simulink model "f_validation_V1_19b"  (R2019b)
settings: Solver=ode4  StartTime=0.0  StopTime=104  FixedStep=0.01  RelTol=1e-3
model workspace (MAT data in the model file):
  x2xx = 0
values from neighbouring files (symbols this model uses):
  KDspd = 0    [frequency_validation.m]
  KIspd = 0    [frequency_validation.m]
  KPspd = 20    [frequency_validation.m]
  PARSa = [ ... (first row only)    [Q_ART_par.m]
  PARSu = zeros(Nu,5)    [Q_ART_par.m]
  Q0 = zeros(Nu+2,1)    [frequency_validation.m]
  QD0 = Q0    [frequency_validation.m]
  v_ref = vconst    (= 5.55555555556)    [frequency_validation.m]
undefined symbols (not defined in the file or in its folder): axle_rate_limit, Lspd, Nspd, Tmc, Uspd
libraries: simulink x2
(part 2 of 3)

== matlab function f_validation_V1_19b/time-domain-test/single-funky-sattyre-nonlinear-variable-crrc/V_tyre ==
  data: q input; Vaa output; qd input
function Vaa = calculate_v_tyre(q, qd)

%%%%%%%%%%%%%%%%%%%%%%%%%%%%%%%%%%%%%%%%%%%%%%%%%%%%%%%%%%%%%%%%%%%%%%%%%
Va = zeros(2, 8); % axle velocities in globals
Vj = zeros(2, 4); % joint velocities in globals
Vaa = Va; % axle velocities in locals
%%%%%%%%%%%%%%%%%%%%%%%%%%%%%%%%%%%%%%%%%%%%%%%%%%%%%%%%%%%%%%%%%%%%%%%%%%
% Parameter given
% M J L xg = mass, moment of inertia, length, cg location measured from rear joint

LL = [11.4, 9.4, 11.4]';
XG = [5.538, 4.757, 11.4 - 5.538]';
XA = [8.9, 7.4, 1.5, 7.9, 1.5, 9.9, 4.0, 2.5]';
KK = [1, 1, 1, 2, 2, 3, 3, 3]';
%%%%%%%%%%%%%%%%%%%%%%%%%%%%%%%%%%%%%%%%%%%%%%%%%%%%%%%%%%%%%%%%%%%%%%%%%%
% Rotation matrix

uu = zeros(2, 3); 
nn = zeros(2, 3); 
for i = 1:3
    c = cos(q(i + 2));
    s = sin(q(i + 2)); 
    uu(:, i) = [c, s]';
    nn(:, i) = [-s, c]';
end
%%%%%%%%%%%%%%%%%%%%%%%%%%%%%%%%%%%%%%%%%%%%%%%%%%%%%%%%%%%%%%%%%%%%%%%%%%
% % from first unit cg to first virtual joint
% 
% l = 11.4;
% b1 = 5.538;
% 
% q = zeros(5,1);
% q(1) = q(1) + (l - b1) * cos(q(3));
% q(2) = q(2) + (l - b1) * sin(q(3));
% 
% qd = zeros(5,1);
% qd(1) = qd(1) + (l - b1) * qd(3) * sin(q(3));
% qd(2) = qd(2) - (l - b1) * qd(3) * cos(q(3));
%%%%%%%%%%%%%%%%%%%%%%%%%%%%%%%%%%%%%%%%%%%%%%%%%%%%%%%%%%%%%%%%%%%%%%%%%%
% calculate v_tyre

Vj(:, 1) = [qd(1), qd(2)]';

for i = 1:3
    Vj(:, i+1) = Vj(:, i) - qd(i + 2) * LL(i) * nn(:, i);
end

for i = 1:8
    Va(:, i) = Vj(:, KK(i) + 1) + qd(KK(i) + 2) * XA(i) * nn(:, KK(i));
    Vax = dot(Va(:, i), uu(:, KK(i)));
    Vay = dot(Va(:, i), nn(:, KK(i)));
    Vaa(:, i) = [Vax; Vay];
end
%%%%%%%%%%%%%%%%%%%%%%%%%%%%%%%%%%%%%%%%%%%%%%%%%%%%%%%%%%%%%%%%%%%%%%%%%%

== matlab function f_validation_V1_19b/time-domain-test/single-general-lineartyre-nonlinear-variable-crrc/qdd ==
  data: M input; C input; Q input; qdd output
function qdd = calculate_qdd(M, C, Q)

qdd = inv(M)*(Q - C);

end

== matlab function f_validation_V1_19b/time-domain-test/single-funky-sattyre-nonlinear-variable-crrc/Fy from slip ==
  data: Alpha output; Steer input; V_tyre input; Fy output
function [Alpha, Fy] = LatForce(Steer, V_tyre)

small = 1e-4;
deg = pi/180;
Fy = zeros(8, 1); 
Alpha = zeros(8, 1); 
Ca = 3065 * 180 / pi;
Sat = Ca * 10 * deg; 

for i = 1:8
    vx = V_tyre(1, i) * cos(Steer(i)) + V_tyre(2, i) * sin(Steer(i));
    vy = -V_tyre(1, i) * sin(Steer(i)) + V_tyre(2, i) * cos(Steer(i));
    if abs(vx) < small
        if abs(vy) < small
            alpha = 0;
            fy = 0.0;
        else
            alpha = 90;
            fy = -Sat * sign(vy);
        end
    else
        alpha = atan2(vy, vx);
        fy = abs(Ca * alpha);
        fy = min(Sat, fy);
        fy = -fy * sign(vy);
    end
    Fy(i) = fy;
    Alpha(i) = alpha;
end

== matlab function f_validation_V1_19b/time-domain-test/double-general-lineartyre-nonlinear-variable-matrix/C ==
  data: q input; qd input; C output
function C = calculate_C(q, qd)

m1 = 11142;
m3 = 11142;
m2 = 7651; 
l_j1j2 = 11.4;
l_j2j3 = 9.4;
l_j1g1 = 5.862; 
l_j2g2 = 4.643; 
l_j3g3 = 5.538; 

psi1 = q(3);
psi2 = q(4);
psi3 = q(5);
xd = qd(1);
yd = qd(2);
psi1d = qd(3);
psi2d = qd(4);
psi3d = qd(5);

C = [0, 0, (l_j1g1*m1 + l_j1j2*(m2 + m3))*cos(psi1)*psi1d, (l_j2g2*m2 + l_j2j3*m3)*cos(psi2)*psi2d, l_j3g3*m3*cos(psi3)*psi3d;
     0, 0, (l_j1g1*m1 + l_j1j2*(m2 + m3))*sin(psi1)*psi1d, (l_j2g2*m2 + l_j2j3*m3)*sin(psi2)*psi2d, l_j3g3*m3*sin(psi3)*psi3d;
     1/2*(l_j1g1*m1 + l_j1j2*(m2 + m3))*cos(psi1)*psi1d, 1/2*(l_j1g1*m1 + l_j1j2*(m2 + m3))*sin(psi1)*psi1d, -1/2*(l_j1g1*m1 + l_j1j2*(m2 + m3))*(xd*cos(psi1)+yd*sin(psi1))+1/2*(l_j2g2*l_j1j2*m2+l_j1j2*l_j2j3*m3)*sin(psi1-psi2)*psi2d+1/2*l_j3g3*l_j1j2*m3*sin(psi1-psi3)*psi3d, (l_j2g2*l_j1j2*m2+l_j1j2*l_j2j3*m3)*sin(psi1-psi2)*(-1/2*psi1d+psi2d), l_j3g3*l_j1j2*m3*sin(psi1-psi3)*(-1/2*psi1d+psi3d);
     1/2*(l_j2g2*m2 + l_j2j3*m3)*cos(psi2)*psi2d, 1/2*(l_j2g2*m2 + l_j2j3*m3)*sin(psi2)*psi2d, (l_j2g2*l_j1j2*m2+l_j1j2*l_j2j3*m3)*sin(psi1-psi2)*(-psi1d+1/2*psi2d), -1/2*(l_j2g2*m2+l_j2j3*m3)*(xd*cos(psi2)+yd*sin(psi2))-1/2*(l_j2g2*l_j1j2*m2+l_j1j2*l_j2j3*m3)*sin(psi1-psi2)*psi1d+1/2*l_j3g3*l_j2j3*m3*sin(psi2-psi3)*psi3d, l_j3g3*l_j2j3*m3*sin(psi2-psi3)*(-1/2*psi2d+psi3d);
     1/2*l_j3g3*m3*cos(psi3)*psi3d, 1/2*l_j3g3*m3*sin(psi3)*psi3d, l_j3g3*l_j1j2*m3*sin(psi1-psi3)*(-psi1d+1/2*psi3d), l_j3g3*l_j2j3*m3*sin(psi2-psi3)*(-psi2d+1/2*psi3d), -1/2*l_j3g3*m3*(xd*cos(psi3)+yd*sin(psi3))-1/2*l_j3g3*l_j1j2*m3*sin(psi1-psi3)*psi1d-1/2*l_j3g3*l_j2j3*m3*sin(psi2-psi3)*psi2d;];

end

== matlab function f_validation_V1_19b/time-domain-test/double-general-lineartyre-nonlinear-variable-matrix/D ==
  data: D output
function D = calculate_D()

d1 = 10000;
d2 = 10000;

delta_kj = eye(3);
dj = [0, d1, d2, 0]';
D = zeros(5);

for k = 1:5
    for l = 1:5
        if k > 2 && l > 2
            if  l == k
                D(k, l) = (1 - delta_kj(1, k-2))*dj(k - 2) + (1 - delta_kj(3, k-2))*dj(k - 1);
            elseif l == k-1
                D(k, l) = -(1 - delta_kj(1, k-2))*dj(k - 2);
            elseif l == k+1
                D(k, l) = -(1 - delta_kj(3, k-2))*dj(k - 1);
            else
                D(k, l) = 0;
            end
        end
    end
end

end

== matlab function f_validation_V1_19b/time-domain-test/double-general-lineartyre-nonlinear-variable-matrix1/qdd ==
  data: M input; C input; D input; qd input; Q input; qdd output
function qdd = calculate_qdd(M, C, D, qd, Q)

qdd = inv(M)*(Q - C * qd - D * qd);

end

== matlab function f_validation_V1_19b/time-domain-test/double-general-lineartyre-nonlinear-variable-matrix/M ==
  data: M output; q input
function M = calculate_M(q)

psi1 = q(3);
psi2 = q(4);
psi3 = q(5);

m1 = 11142;
m3 = 11142;
m2 = 7651; 
l_j1j2 = 11.4;
l_j2j3 = 9.4;
l_j1g1 = 5.862; 
l_j2g2 = 4.643; 
l_j3g3 = 5.538; 
iz1 = 143570; 
iz3 = 143570; 
iz2 = 37800;

l_kj = [l_j1g1, l_j1j2, l_j1j2;
             0, l_j2g2, l_j2j3;
             0,      0, l_j3g3;];
delta_kj = eye(3);
Jc = zeros(3, 5, 3);
for j = 1:3
    Jc(:, :, j) = [1, 0,  l_kj(1, j) * sin(psi1),  l_kj(2, j) * sin(psi2),  l_kj(3, j) * sin(psi3);
          0, 1, -l_kj(1, j) * cos(psi1), -l_kj(2, j) * cos(psi2), -l_kj(3, j) * cos(psi3);
          0, 0,          delta_kj(1, j),          delta_kj(2, j),          delta_kj(3, j);];
end

mj = [m1, m2, m3]';
izj = [iz1, iz2, iz3]';
Mj = zeros(3, 3, 3);
for j = 1:3
    Mj(:, :, j) = diag([mj(j), mj(j), izj(j)]);
end

M = zeros(5, 5);
for j = 1:3
    M = M + Jc(:, :, j)' * Mj(:, :, j) * Jc(:, :, j);
end

end

== matlab function f_validation_V1_19b/time-domain-test/double-general-lineartyre-nonlinear-variable-matrix/Tau_tire ==
  data: q input; qd input; delta input; Fx input; Tau_tire output; Alpha output
function [Tau_tire, Alpha] = calculate_Tau_tire(q, qd, delta, Fx)

% coefficient

l_j1j2 = 11.4;
l_j2j3 = 9.4;
l_j1a1 = 2.5;
l_j1a2 = 4;
l_j1a3 = 9.9;
l_j2a4 = 1.5;
l_j2a5 = 7.9;
l_j3a6 = 1.5;
l_j3a7 = 7.4;
l_j3a8 = 8.9;
h11 = 0.9625;
h12 = 0.9625;
h13 = 0.98;
h21 = 0.98; 
h22 = 0.98;
h31 = 0.98;
h32 = 0.9625;
h33 = 0.9625;
ca1 = 3065 * 180 / pi;
ca2 = 3065 * 180 / pi;
ca3 = 3065 * 180 / pi;
ca4 = 3065 * 180 / pi;
ca5 = 3065 * 180 / pi;
ca6 = 3065 * 180 / pi;
ca7 = 3065 * 180 / pi;
ca8 = 3065 * 180 / pi;

x = q(1);
y = q(2);
psi1 = q(3);
psi2 = q(4);
psi3 = q(5);
xd = qd(1);
yd = qd(2);
psi1d = qd(3);
psi2d = qd(4);
psi3d = qd(5);

psij = [psi1, psi2, psi3]';
Rot_w2v = zeros(2, 2, 3);
for i = 1:3
    Rot_w2v(:, :, i) = [cos(psij(i)), -sin(psij(i));
                        sin(psij(i)), cos(psij(i));];
end

Rot_v2t = zeros(2, 2, 8);
for i = 1:8
    Rot_v2t(:, :, i) = [cos(delta(i)), -sin(delta(i));
                        sin(delta(i)), cos(delta(i));];
end

xj = zeros(3, 1);
yj = zeros(3, 1);
xj(1) = x;
yj(1) = y;
xj(2) = x - l_j1j2*cos(psi1);
yj(2) = y - l_j1j2*sin(psi1);
xj(3) = x - l_j1j2*cos(psi1) - l_j2j3*cos(psi2);
yj(3) = y - l_j1j2*sin(psi1) - l_j2j3*sin(psi2);

u = zeros(2, 3);
n = zeros(2, 3);
for i = 1:3
    u(:, i)=[cos(q(i + 2)), sin(q(i + 2))]';
    n(:, i)=[-sin(q(i + 2)), cos(q(i + 2))]';
end

IU = [1, 1, 1, 2, 2, 3, 3, 3]';
l_ja = [l_j1a1, l_j1a2, l_j1a3, l_j2a4, l_j2a5, l_j3a6, l_j3a7, l_j3a8]';
ha = [h11, h12, h13, h21, h22, h31, h32, h33]';

L_long1 = [cos(psi1), cos(psi1), cos(psi1), cos(psi2), cos(psi2), cos(psi3), cos(psi3), cos(psi3);
           sin(psi1), sin(psi1), sin(psi1), sin(psi2), sin(psi2), sin(psi3), sin(psi3), sin(psi3);
           -h11, -h12, -h13, l_j1j2*sin(psi1-psi2), l_j1j2*sin(psi1-psi2), l_j1j2*sin(psi1-psi3), l_j1j2*sin(psi1-psi3), l_j1j2*sin(psi1-psi3);
           0, 0, 0, -h21, -h22, l_j2j3*sin(psi2-psi3), l_j2j3*sin(psi2-psi3), l_j2j3*sin(psi2-psi3);
           0, 0, 0, 0, 0, -h31, -h32, -h33;];

L_long2 = [cos(psi1), cos(psi1), cos(psi1), cos(psi2), cos(psi2), cos(psi3), cos(psi3), cos(psi3);
           sin(psi1), sin(psi1), sin(psi1), sin(psi2), sin(psi2), sin(psi3), sin(psi3), sin(psi3);
           h11, h12, h13, l_j1j2*sin(psi1-psi2), l_j1j2*sin(psi1-psi2), l_j1j2*sin(psi1-psi3), l_j1j2*sin(psi1-psi3), l_j1j2*sin(psi1-psi3);
           0, 0, 0, h21, h22, l_j2j3*sin(psi2-psi3), l_j2j3*sin(psi2-psi3), l_j2j3*sin(psi2-psi3);
           0, 0, 0, 0, 0, h31, h32, h33;];

L_lat1 = [-sin(psi1), -sin(psi1), -sin(psi1), -sin(psi2), -sin(psi2), -sin(psi3), -sin(psi3), -sin(psi3);
          cos(psi1), cos(psi1), cos(psi1), cos(psi2), cos(psi2), cos(psi3), cos(psi3), cos(psi3);
          -l_j1a1, -l_j1a2, -l_j1a3, -l_j1j2*cos(psi1-psi2), -l_j1j2*cos(psi1-psi2), -l_j1j2*cos(psi1-psi3), -l_j1j2*cos(psi1-psi3), -l_j1j2*cos(psi1-psi3);
          0, 0, 0, -l_j2a4, -l_j2a5, -l_j2j3*cos(psi2-psi3), -l_j2j3*cos(psi2-psi3), -l_j2j3*cos(psi2-psi3);
          0, 0, 0, 0, 0, -l_j3a6, -l_j3a7, -l_j3a8;];

L_lat2 = [-sin(psi1), -sin(psi1), -sin(psi1), -sin(psi2), -sin(psi2), -sin(psi3), -sin(psi3), -sin(psi3);
          cos(psi1), cos(psi1), cos(psi1), cos(psi2), cos(psi2), cos(psi3), cos(psi3), cos(psi3);
          -l_j1a1, -l_j1a2, -l_j1a3, -l_j1j2*cos(psi1-psi2), -l_j1j2*cos(psi1-psi2), -l_j1j2*cos(psi1-psi3), -l_j1j2*cos(psi1-psi3), -l_j1j2*cos(psi1-psi3);
          0, 0, 0, -l_j2a4, -l_j2a5, -l_j2j3*cos(psi2-psi3), -l_j2j3*cos(psi2-psi3), -l_j2j3*cos(psi2-psi3);
          0, 0, 0, 0, 0, -l_j3a6, -l_j3a7, -l_j3a8;];

Delta_c = zeros(8, 8);
Delta_s = zeros(8, 8);
for i = 1:8
    Delta_c(i, i) = cos(delta(i));
    Delta_s(i, i) = sin(delta(i));
end

vxj = zeros(3, 1);
vyj = zeros(3, 1);
vxj(1) = xd;
vyj(1) = yd;
vxj(2) = xd + l_j1j2*sin(psi1)*psi1d;
vyj(2) = yd - l_j1j2*cos(psi1)*psi1d;
vxj(3) = xd + l_j1j2*sin(psi1)*psi1d + l_j2j3*sin(psi2)*psi2d;
vyj(3) = yd - l_j1j2*cos(psi1)*psi1d - l_j2j3*cos(psi2)*psi2d;
va1 = zeros(2, 8);
va2 = zeros(2, 8);
psidj = [psi1d, psi2d, psi3d]';
for i = 1:8
    va1(:, i) = [vxj(IU(i)); vyj(IU(i))] - n(:, IU(i))*l_ja(i)*psidj(IU(i)) + (-1)*u(:, IU(i))*ha(i)*psidj(IU(i));
    va2(:, i) = [vxj(IU(i)); vyj(IU(i))] - n(:, IU(i))*l_ja(i)*psidj(IU(i)) + u(:, IU(i))*ha(i)*psidj(IU(i));
end

va1_v = zeros(2, 8);
va2_v = zeros(2, 8);
for i = 1:8
    va1_v(:, i) = inv(Rot_w2v(:, :, IU(i)))*va1(:, i);
    va2_v(:, i) = inv(Rot_w2v(:, :, IU(i)))*va2(:, i);
end

beta1 = zeros(8, 1);
beta2 = zeros(8, 1);
for i = 1:8
    beta1(i) = atan2(va1_v(2, i), va1_v(1, i));
    beta2(i) = atan2(va2_v(2, i), va2_v(1, i));
end

ca = [ca1, ca2, ca3, ca4, ca5, ca6, ca7, ca8]';
Ca = diag(ca);

Tau_tire = L_long1 * (Delta_c * Fx / 2 - Delta_s * Ca * (delta - beta1)) ...
         + L_long2 * (Delta_c * Fx / 2 - Delta_s * Ca * (delta - beta2)) ...
         + L_lat1 * (Delta_s * Fx / 2 + Delta_c * Ca * (delta - beta1)) ...
         + L_lat2 * (Delta_s * Fx / 2 + Delta_c * Ca * (delta - beta2));

beta = (beta1 + beta2) / 2;
Alpha = delta - beta;

end

== matlab function f_validation_V1_19b/time-domain-test/double-general-lineartyre-nonlinear-variable-matrix/qdd ==
  data: M input; C input; D input; qd input; Q input; qdd output
function qdd = calculate_qdd(M, C, D, qd, Q)

qdd = inv(M)*(Q - C * qd - D * qd);

end

== matlab function f_validation_V1_19b/time-domain-test/single-general-lineartyre-nonlinear-variable-matrix/C ==
  data: q input; qd input; C output
function C = calculate_C(q, qd)

m1 = 11142;
m3 = 11142;
m2 = 7651; 
l_j1j2 = 11.4;
l_j2j3 = 9.4;
l_j1g1 = 5.862; 
l_j2g2 = 4.643; 
l_j3g3 = 5.538; 

psi1 = q(3);
psi2 = q(4);
psi3 = q(5);
xd = qd(1);
yd = qd(2);
psi1d = qd(3);
psi2d = qd(4);
psi3d = qd(5);

C = [0, 0, (l_j1g1*m1 + l_j1j2*(m2 + m3))*cos(psi1)*psi1d, (l_j2g2*m2 + l_j2j3*m3)*cos(psi2)*psi2d, l_j3g3*m3*cos(psi3)*psi3d;
     0, 0, (l_j1g1*m1 + l_j1j2*(m2 + m3))*sin(psi1)*psi1d, (l_j2g2*m2 + l_j2j3*m3)*sin(psi2)*psi2d, l_j3g3*m3*sin(psi3)*psi3d;
     1/2*(l_j1g1*m1 + l_j1j2*(m2 + m3))*cos(psi1)*psi1d, 1/2*(l_j1g1*m1 + l_j1j2*(m2 + m3))*sin(psi1)*psi1d, -1/2*(l_j1g1*m1 + l_j1j2*(m2 + m3))*(xd*cos(psi1)+yd*sin(psi1))+1/2*(l_j2g2*l_j1j2*m2+l_j1j2*l_j2j3*m3)*sin(psi1-psi2)*psi2d+1/2*l_j3g3*l_j1j2*m3*sin(psi1-psi3)*psi3d, (l_j2g2*l_j1j2*m2+l_j1j2*l_j2j3*m3)*sin(psi1-psi2)*(-1/2*psi1d+psi2d), l_j3g3*l_j1j2*m3*sin(psi1-psi3)*(-1/2*psi1d+psi3d);
     1/2*(l_j2g2*m2 + l_j2j3*m3)*cos(psi2)*psi2d, 1/2*(l_j2g2*m2 + l_j2j3*m3)*sin(psi2)*psi2d, (l_j2g2*l_j1j2*m2+l_j1j2*l_j2j3*m3)*sin(psi1-psi2)*(-psi1d+1/2*psi2d), -1/2*(l_j2g2*m2+l_j2j3*m3)*(xd*cos(psi2)+yd*sin(psi2))-1/2*(l_j2g2*l_j1j2*m2+l_j1j2*l_j2j3*m3)*sin(psi1-psi2)*psi1d+1/2*l_j3g3*l_j2j3*m3*sin(psi2-psi3)*psi3d, l_j3g3*l_j2j3*m3*sin(psi2-psi3)*(-1/2*psi2d+psi3d);
     1/2*l_j3g3*m3*cos(psi3)*psi3d, 1/2*l_j3g3*m3*sin(psi3)*psi3d, l_j3g3*l_j1j2*m3*sin(psi1-psi3)*(-psi1d+1/2*psi3d), l_j3g3*l_j2j3*m3*sin(psi2-psi3)*(-psi2d+1/2*psi3d), -1/2*l_j3g3*m3*(xd*cos(psi3)+yd*sin(psi3))-1/2*l_j3g3*l_j1j2*m3*sin(psi1-psi3)*psi1d-1/2*l_j3g3*l_j2j3*m3*sin(psi2-psi3)*psi2d;];

end

== matlab function f_validation_V1_19b/time-domain-test/single-general-lineartyre-nonlinear-variable-matrix/D ==
  data: D output
function D = calculate_D()

d1 = 0;
d2 = 0;

delta_kj = eye(3);
dj = [0, d1, d2, 0]';
D = zeros(5);

for k = 1:5
    for l = 1:5
        if k > 2 && l > 2
            if  l == k
                D(k, l) = (1 - delta_kj(1, k-2))*dj(k - 2) + (1 - delta_kj(3, k-2))*dj(k - 1);
            elseif l == k-1
                D(k, l) = -(1 - delta_kj(1, k-2))*dj(k - 2);
            elseif l == k+1
                D(k, l) = -(1 - delta_kj(3, k-2))*dj(k - 1);
            else
                D(k, l) = 0;
            end
        end
    end
end

end

== matlab function f_validation_V1_19b/time-domain-test/single-general-lineartyre-nonlinear-variable-matrix/M ==
  data: M output; q input
function M = calculate_M(q)

psi1 = q(3);
psi2 = q(4);
psi3 = q(5);

m1 = 11142;
m3 = 11142;
m2 = 7651; 
l_j1j2 = 11.4;
l_j2j3 = 9.4;
l_j1g1 = 5.862; 
l_j2g2 = 4.643; 
l_j3g3 = 5.538; 
iz1 = 143570; 
iz3 = 143570; 
iz2 = 37800;

l_kj = [l_j1g1, l_j1j2, l_j1j2;
             0, l_j2g2, l_j2j3;
             0,      0, l_j3g3;];
delta_kj = eye(3);
Jc = zeros(3, 5, 3);
for j = 1:3
    Jc(:, :, j) = [1, 0,  l_kj(1, j) * sin(psi1),  l_kj(2, j) * sin(psi2),  l_kj(3, j) * sin(psi3);
          0, 1, -l_kj(1, j) * cos(psi1), -l_kj(2, j) * cos(psi2), -l_kj(3, j) * cos(psi3);
          0, 0,          delta_kj(1, j),          delta_kj(2, j),          delta_kj(3, j);];
end

mj = [m1, m2, m3]';
izj = [iz1, iz2, iz3]';
Mj = zeros(3, 3, 3);
for j = 1:3
    Mj(:, :, j) = diag([mj(j), mj(j), izj(j)]);
end

M = zeros(5, 5);
for j = 1:3
    M = M + Jc(:, :, j)' * Mj(:, :, j) * Jc(:, :, j);
end

end

== matlab function f_validation_V1_19b/time-domain-test/single-general-lineartyre-nonlinear-variable-matrix/Tau_tire ==
  data: q input; qd input; delta input; Fx input; Tau_tire output; Alpha output
function [Tau_tire, Alpha] = calculate_Tau_tire(q, qd, delta, Fx)

% coefficient

l_j1j2 = 11.4;
l_j2j3 = 9.4;
l_j1a1 = 2.5;
l_j1a2 = 4;
l_j1a3 = 9.9;
l_j2a4 = 1.5;
l_j2a5 = 7.9;
l_j3a6 = 1.5;
l_j3a7 = 7.4;
l_j3a8 = 8.9;

LL = [l_j1j2, l_j2j3, l_j1j2]';
JA = [l_j1a1, l_j1a2, l_j1a3, l_j2a4, l_j2a5, l_j3a6, l_j3a7, l_j3a8]';
XA = [l_j1j2, l_j1j2, l_j1j2, l_j2j3, l_j2j3, l_j1j2, l_j1j2, l_j1j2]' - JA;
IU = [1, 1, 1, 2, 2, 3, 3, 3]';

Ca = [3065 * 180 / pi, 3065 * 180 / pi, 3065 * 180 / pi, 3065 * 180 / pi, 3065 * 180 / pi, 3065 * 180 / pi, 3065 * 180 / pi, 3065 * 180 / pi]';

uu = zeros(2, 3);
nn = zeros(2, 3);
for i = 1:3
    uu(:, i)=[cos(q(i + 2)), sin(q(i + 2))]';
    nn(:, i)=[-sin(q(i + 2)), cos(q(i + 2))]';
end

psi1 = q(3);
psi2 = q(4);
psi3 = q(5);
xd = qd(1);
yd = qd(2);
psi1d = qd(3);
psi2d = qd(4);
psi3d = qd(5);
psij = [psi1, psi2, psi3]';
l_ja = [l_j1a1, l_j1a2, l_j1a3, l_j2a4, l_j2a5, l_j3a6, l_j3a7, l_j3a8]';

Rot_w2v = zeros(2, 2, 3);
for i = 1:3
    Rot_w2v(:, :, i) = [cos(psij(i)), -sin(psij(i));
                        sin(psij(i)), cos(psij(i));];
end

Rot_v2t = zeros(2, 2, 8);
for i = 1:8
    Rot_v2t(:, :, i) = [cos(delta(i)), -sin(delta(i));
                        sin(delta(i)), cos(delta(i));];
end

vxj = zeros(3, 1);
vyj = zeros(3, 1);
vxj(1) = xd;
vyj(1) = yd;
vxj(2) = xd + l_j1j2*sin(psi1)*psi1d;
vyj(2) = yd - l_j1j2*cos(psi1)*psi1d;
vxj(3) = xd + l_j1j2*sin(psi1)*psi1d + l_j2j3*sin(psi2)*psi2d;
vyj(3) = yd - l_j1j2*cos(psi1)*psi1d - l_j2j3*cos(psi2)*psi2d;
va = zeros(2, 8);
psidj = [psi1d, psi2d, psi3d]';
for i = 1:8
    va(:, i) = [vxj(IU(i)); vyj(IU(i))] - nn(:, IU(i))*l_ja(i)*psidj(IU(i));
end

Va_v = zeros(2, 8);  % axle velocities in locals
for i = 1:8
    Va_v(:, i) = inv(Rot_w2v(:, :, IU(i)))*va(:, i);
end

Fy = zeros(8, 1); 
Alpha = zeros(8, 1); 

beta = zeros(8, 1);
for i = 1:8
    beta(i) = atan2(Va_v(2, i), Va_v(1, i));
end

Vx_t = zeros(8, 1);
Vy_t = zeros(8, 1);
for i = 1:8
    Vx_t(i) = Va_v(1, i) * cos(delta(i)) + Va_v(2, i) * sin(delta(i));
    Vy_t(i) = -Va_v(1, i) * sin(delta(i)) + Va_v(2, i) * cos(delta(i));
end

for i = 1:8
    Alpha(i) = delta(i) - beta(i);
%     Fy(i) = -sign(Vy_t(i)) * Ca(i) * abs(Alpha(i));
    Fy(i) = Ca(i) * Alpha(i);
end

% for i = 1:8
%     vx = Va_v(1, i) * cos(delta(i)) + Va_v(2, i) * sin(delta(i));
%     vy = -Va_v(1, i) * sin(delta(i)) + Va_v(2, i) * cos(delta(i));
%     alpha = atan2(vy, vx);
%     Alpha(i) = alpha;
%     Fy(i) = -abs(Ca(i) * alpha) * sign(vy);
% end

L_long = [cos(psi1), cos(psi1), cos(psi1), cos(psi2), cos(psi2), cos(psi3), cos(psi3), cos(psi3);
           sin(psi1), sin(psi1), sin(psi1), sin(psi2), sin(psi2), sin(psi3), sin(psi3), sin(psi3);
           0, 0, 0, l_j1j2*sin(psi1-psi2), l_j1j2*sin(psi1-psi2), l_j1j2*sin(psi1-psi3), l_j1j2*sin(psi1-psi3), l_j1j2*sin(psi1-psi3);
           0, 0, 0, 0, 0, l_j2j3*sin(psi2-psi3), l_j2j3*sin(psi2-psi3), l_j2j3*sin(psi2-psi3);
           0, 0, 0, 0, 0, 0, 0, 0;];

L_lat = [-sin(psi1), -sin(psi1), -sin(psi1), -sin(psi2), -sin(psi2), -sin(psi3), -sin(psi3), -sin(psi3);
          cos(psi1), cos(psi1), cos(psi1), cos(psi2), cos(psi2), cos(psi3), cos(psi3), cos(psi3);
          -l_j1a1, -l_j1a2, -l_j1a3, -l_j1j2*cos(psi1-psi2), -l_j1j2*cos(psi1-psi2), -l_j1j2*cos(psi1-psi3), -l_j1j2*cos(psi1-psi3), -l_j1j2*cos(psi1-psi3);
          0, 0, 0, -l_j2a4, -l_j2a5, -l_j2j3*cos(psi2-psi3), -l_j2j3*cos(psi2-psi3), -l_j2j3*cos(psi2-psi3);
          0, 0, 0, 0, 0, -l_j3a6, -l_j3a7, -l_j3a8;];

Delta_c = zeros(8, 8);
Delta_s = zeros(8, 8);
for i = 1:8
    Delta_c(i, i) = cos(delta(i));
    Delta_s(i, i) = sin(delta(i));
end

Tau_tire = L_long * (Delta_c * Fx - Delta_s * Fy) + L_lat * (Delta_s * Fx + Delta_c * Fy);

end

== matlab function f_validation_V1_19b/time-domain-test/single-general-lineartyre-nonlinear-variable-matrix/qdd ==
  data: M input; C input; D input; qd input; Q input; qdd output
function qdd = calculate_qdd(M, C, D, qd, Q)

qdd = inv(M)*(Q - C * qd - D * qd);

end

== matlab function f_validation_V1_19b/time-domain-test/double-general-lineartyre-nonlinear-constant-matrix/C ==
  data: q input; qd input; C output
function C = calculate_C(q, qd)

m1 = 11142;
m3 = 11142;
m2 = 7651; 
l_j1j2 = 11.4;
l_j2j3 = 9.4;
l_j1g1 = 5.862; 
l_j2g2 = 4.643; 
l_j3g3 = 5.538; 

psi1 = q(3);
psi2 = q(4);
psi3 = q(5);
xd = qd(1);
yd = qd(2);
psi1d = qd(3);
psi2d = qd(4);
psi3d = qd(5);

C = [0, 0, (l_j1g1*m1 + l_j1j2*(m2 + m3))*cos(psi1)*psi1d, (l_j2g2*m2 + l_j2j3*m3)*cos(psi2)*psi2d, l_j3g3*m3*cos(psi3)*psi3d;
     0, 0, (l_j1g1*m1 + l_j1j2*(m2 + m3))*sin(psi1)*psi1d, (l_j2g2*m2 + l_j2j3*m3)*sin(psi2)*psi2d, l_j3g3*m3*sin(psi3)*psi3d;
     1/2*(l_j1g1*m1 + l_j1j2*(m2 + m3))*cos(psi1)*psi1d, 1/2*(l_j1g1*m1 + l_j1j2*(m2 + m3))*sin(psi1)*psi1d, -1/2*(l_j1g1*m1 + l_j1j2*(m2 + m3))*(xd*cos(psi1)+yd*sin(psi1))+1/2*(l_j2g2*l_j1j2*m2+l_j1j2*l_j2j3*m3)*sin(psi1-psi2)*psi2d+1/2*l_j3g3*l_j1j2*m3*sin(psi1-psi3)*psi3d, (l_j2g2*l_j1j2*m2+l_j1j2*l_j2j3*m3)*sin(psi1-psi2)*(-1/2*psi1d+psi2d), l_j3g3*l_j1j2*m3*sin(psi1-psi3)*(-1/2*psi1d+psi3d);
     1/2*(l_j2g2*m2 + l_j2j3*m3)*cos(psi2)*psi2d, 1/2*(l_j2g2*m2 + l_j2j3*m3)*sin(psi2)*psi2d, (l_j2g2*l_j1j2*m2+l_j1j2*l_j2j3*m3)*sin(psi1-psi2)*(-psi1d+1/2*psi2d), -1/2*(l_j2g2*m2+l_j2j3*m3)*(xd*cos(psi2)+yd*sin(psi2))-1/2*(l_j2g2*l_j1j2*m2+l_j1j2*l_j2j3*m3)*sin(psi1-psi2)*psi1d+1/2*l_j3g3*l_j2j3*m3*sin(psi2-psi3)*psi3d, l_j3g3*l_j2j3*m3*sin(psi2-psi3)*(-1/2*psi2d+psi3d);
     1/2*l_j3g3*m3*cos(psi3)*psi3d, 1/2*l_j3g3*m3*sin(psi3)*psi3d, l_j3g3*l_j1j2*m3*sin(psi1-psi3)*(-psi1d+1/2*psi3d), l_j3g3*l_j2j3*m3*sin(psi2-psi3)*(-psi2d+1/2*psi3d), -1/2*l_j3g3*m3*(xd*cos(psi3)+yd*sin(psi3))-1/2*l_j3g3*l_j1j2*m3*sin(psi1-psi3)*psi1d-1/2*l_j3g3*l_j2j3*m3*sin(psi2-psi3)*psi2d;];

c33 = -1/2*(l_j1g1*m1 + l_j1j2*(m2 + m3)) * ( (xd*cos(psi1)-yd*sin(psi1)-xd) * cos(psi1) + (xd*sin(psi1)+yd*cos(psi1)-yd) * sin(psi1) );
c44 = -1/2*(l_j2g2*m2 + l_j2j3*m3) * ( (xd*cos(psi1)-yd*sin(psi1)-xd) * cos(psi2) + (xd*sin(psi1)+yd*cos(psi1)-yd) * sin(psi2) );
c55 = -1/2*l_j3g3*m3 * ( (xd*cos(psi1)-yd*sin(psi1)-xd) * cos(psi3) + (xd*sin(psi1)+yd*cos(psi1)-yd) * sin(psi3) );
C_wv = [0, 0, 0, 0, 0;
        0, 0 ,0, 0, 0;
        0, 0, c33, 0, 0;
        0, 0, 0, c44, 0;
        0, 0, 0, 0, c55;];

C = C + C_wv;

end

== matlab function f_validation_V1_19b/time-domain-test/double-general-lineartyre-nonlinear-constant-matrix/Cv ==
  data: M input; C input; Cv output; Twv input; Tdwv input
function Cv = calculate_Mv(M, C, Twv, Tdwv)

Cv = Twv'*C*Twv + Twv'*M*Tdwv;

end

== matlab function f_validation_V1_19b/time-domain-test/double-general-lineartyre-nonlinear-constant-matrix/D ==
  data: D output
function D = calculate_D()

d1 = 10000;
d2 = 10000;

delta_kj = eye(3);
dj = [0, d1, d2, 0]';
D = zeros(5);

for k = 1:5
    for l = 1:5
        if k > 2 && l > 2
            if  l == k
                D(k, l) = (1 - delta_kj(1, k-2))*dj(k - 2) + (1 - delta_kj(3, k-2))*dj(k - 1);
            elseif l == k-1
                D(k, l) = -(1 - delta_kj(1, k-2))*dj(k - 2);
            elseif l == k+1
                D(k, l) = -(1 - delta_kj(3, k-2))*dj(k - 1);
            else
                D(k, l) = 0;
            end
        end
    end
end

end

== matlab function f_validation_V1_19b/time-domain-test/double-general-lineartyre-nonlinear-constant-matrix/Dv ==
  data: D input; Dv output; Twv input
function Dv = calculate_Mv(D, Twv)

Dv = Twv'*D*Twv;

end

== matlab function f_validation_V1_19b/time-domain-test/double-general-lineartyre-nonlinear-constant-matrix/M ==
  data: M output; q input
function M = calculate_M(q)

psi1 = q(3);
psi2 = q(4);
psi3 = q(5);

m1 = 11142;
m3 = 11142;
m2 = 7651; 
l_j1j2 = 11.4;
l_j2j3 = 9.4;
l_j1g1 = 5.862; 
l_j2g2 = 4.643; 
l_j3g3 = 5.538; 
iz1 = 143570; 
iz3 = 143570; 
iz2 = 37800;

l_kj = [l_j1g1, l_j1j2, l_j1j2;
             0, l_j2g2, l_j2j3;
             0,      0, l_j3g3;];
delta_kj = eye(3);
Jc = zeros(3, 5, 3);
for j = 1:3
    Jc(:, :, j) = [1, 0,  l_kj(1, j) * sin(psi1),  l_kj(2, j) * sin(psi2),  l_kj(3, j) * sin(psi3);
          0, 1, -l_kj(1, j) * cos(psi1), -l_kj(2, j) * cos(psi2), -l_kj(3, j) * cos(psi3);
          0, 0,          delta_kj(1, j),          delta_kj(2, j),          delta_kj(3, j);];
end

mj = [m1, m2, m3]';
izj = [iz1, iz2, iz3]';
Mj = zeros(3, 3, 3);
for j = 1:3
    Mj(:, :, j) = diag([mj(j), mj(j), izj(j)]);
end

M = zeros(5, 5);
for j = 1:3
    M = M + Jc(:, :, j)' * Mj(:, :, j) * Jc(:, :, j);
end

end

== matlab function f_validation_V1_19b/time-domain-test/double-general-lineartyre-nonlinear-constant-matrix/Mv ==
  data: M input; Mv output; Twv input
function Mv = calculate_Mv(M, Twv)

Mv = Twv'*M*Twv;

end

== matlab function f_validation_V1_19b/time-domain-test/double-general-lineartyre-nonlinear-constant-matrix/Tau_tire_v ==
  data: Tau_tire output; Alpha output; q input; qd input; Twv input; delta input
function [Tau_tire, Alpha] = calculate_Tau_tire(q, qd, Twv, delta)

% coefficient

l_j1j2 = 11.4;
l_j2j3 = 9.4;
l_j1a1 = 2.5;
l_j1a2 = 4;
l_j1a3 = 9.9;
l_j2a4 = 1.5;
l_j2a5 = 7.9;
l_j3a6 = 1.5;
l_j3a7 = 7.4;
l_j3a8 = 8.9;
h11 = 0.9625;
h12 = 0.9625;
h13 = 0.98;
h21 = 0.98; 
h22 = 0.98;
h31 = 0.98;
h32 = 0.9625;
h33 = 0.9625;
ca1 = 3065 * 180 / pi;
ca2 = 3065 * 180 / pi;
ca3 = 3065 * 180 / pi;
ca4 = 3065 * 180 / pi;
ca5 = 3065 * 180 / pi;
ca6 = 3065 * 180 / pi;
ca7 = 3065 * 180 / pi;
ca8 = 3065 * 180 / pi;
% ca1 = 400e3;
% ca2 = 400e3;
% ca3 = 400e3;
% ca4 = 400e3;
% ca5 = 400e3;
% ca6 = 400e3;
% ca7 = 400e3;
% ca8 = 400e3;

x = q(1);
y = q(2);
psi1 = q(3);
psi2 = q(4);
psi3 = q(5);
xd = qd(1);
yd = qd(2);
psi1d = qd(3);
psi2d = qd(4);
psi3d = qd(5);

psij = [psi1, psi2, psi3]';
Rot_w2v = zeros(2, 2, 3);
for i = 1:3
    Rot_w2v(:, :, i) = [cos(psij(i)), -sin(psij(i));
                        sin(psij(i)), cos(psij(i));];
end

Rot_v2t = zeros(2, 2, 8);
for i = 1:8
    Rot_v2t(:, :, i) = [cos(delta(i)), -sin(delta(i));
                        sin(delta(i)), cos(delta(i));];
end

xj = zeros(3, 1);
yj = zeros(3, 1);
xj(1) = x;
yj(1) = y;
xj(2) = x - l_j1j2*cos(psi1);
yj(2) = y - l_j1j2*sin(psi1);
xj(3) = x - l_j1j2*cos(psi1) - l_j2j3*cos(psi2);
yj(3) = y - l_j1j2*sin(psi1) - l_j2j3*sin(psi2);

u = zeros(2, 3);
n = zeros(2, 3);
for i = 1:3
    u(:, i)=[cos(q(i + 2)), sin(q(i + 2))]';
    n(:, i)=[-sin(q(i + 2)), cos(q(i + 2))]';
end

IU = [1, 1, 1, 2, 2, 3, 3, 3]';
l_ja = [l_j1a1, l_j1a2, l_j1a3, l_j2a4, l_j2a5, l_j3a6, l_j3a7, l_j3a8]';
ha = [h11, h12, h13, h21, h22, h31, h32, h33]';

L_long1 = [cos(psi1), cos(psi1), cos(psi1), cos(psi2), cos(psi2), cos(psi3), cos(psi3), cos(psi3);
           sin(psi1), sin(psi1), sin(psi1), sin(psi2), sin(psi2), sin(psi3), sin(psi3), sin(psi3);
           -h11, -h12, -h13, l_j1j2*sin(psi1-psi2), l_j1j2*sin(psi1-psi2), l_j1j2*sin(psi1-psi3), l_j1j2*sin(psi1-psi3), l_j1j2*sin(psi1-psi3);
           0, 0, 0, -h21, -h22, l_j2j3*sin(psi2-psi3), l_j2j3*sin(psi2-psi3), l_j2j3*sin(psi2-psi3);
           0, 0, 0, 0, 0, -h31, -h32, -h33;];

L_long2 = [cos(psi1), cos(psi1), cos(psi1), cos(psi2), cos(psi2), cos(psi3), cos(psi3), cos(psi3);
           sin(psi1), sin(psi1), sin(psi1), sin(psi2), sin(psi2), sin(psi3), sin(psi3), sin(psi3);
           h11, h12, h13, l_j1j2*sin(psi1-psi2), l_j1j2*sin(psi1-psi2), l_j1j2*sin(psi1-psi3), l_j1j2*sin(psi1-psi3), l_j1j2*sin(psi1-psi3);
           0, 0, 0, h21, h22, l_j2j3*sin(psi2-psi3), l_j2j3*sin(psi2-psi3), l_j2j3*sin(psi2-psi3);
           0, 0, 0, 0, 0, h31, h32, h33;];

L_lat1 = [-sin(psi1), -sin(psi1), -sin(psi1), -sin(psi2), -sin(psi2), -sin(psi3), -sin(psi3), -sin(psi3);
          cos(psi1), cos(psi1), cos(psi1), cos(psi2), cos(psi2), cos(psi3), cos(psi3), cos(psi3);
          -l_j1a1, -l_j1a2, -l_j1a3, -l_j1j2*cos(psi1-psi2), -l_j1j2*cos(psi1-psi2), -l_j1j2*cos(psi1-psi3), -l_j1j2*cos(psi1-psi3), -l_j1j2*cos(psi1-psi3);
          0, 0, 0, -l_j2a4, -l_j2a5, -l_j2j3*cos(psi2-psi3), -l_j2j3*cos(psi2-psi3), -l_j2j3*cos(psi2-psi3);
          0, 0, 0, 0, 0, -l_j3a6, -l_j3a7, -l_j3a8;];

L_lat2 = [-sin(psi1), -sin(psi1), -sin(psi1), -sin(psi2), -sin(psi2), -sin(psi3), -sin(psi3), -sin(psi3);
          cos(psi1), cos(psi1), cos(psi1), cos(psi2), cos(psi2), cos(psi3), cos(psi3), cos(psi3);
          -l_j1a1, -l_j1a2, -l_j1a3, -l_j1j2*cos(psi1-psi2), -l_j1j2*cos(psi1-psi2), -l_j1j2*cos(psi1-psi3), -l_j1j2*cos(psi1-psi3), -l_j1j2*cos(psi1-psi3);
          0, 0, 0, -l_j2a4, -l_j2a5, -l_j2j3*cos(psi2-psi3), -l_j2j3*cos(psi2-psi3), -l_j2j3*cos(psi2-psi3);
          0, 0, 0, 0, 0, -l_j3a6, -l_j3a7, -l_j3a8;];

Delta_c = zeros(8, 8);
Delta_s = zeros(8, 8);
for i = 1:8
    Delta_c(i, i) = cos(delta(i));
    Delta_s(i, i) = sin(delta(i));
end

vxj = zeros(3, 1);
vyj = zeros(3, 1);
vxj(1) = xd;
vyj(1) = yd;
vxj(2) = xd + l_j1j2*sin(psi1)*psi1d;
vyj(2) = yd - l_j1j2*cos(psi1)*psi1d;
vxj(3) = xd + l_j1j2*sin(psi1)*psi1d + l_j2j3*sin(psi2)*psi2d;
vyj(3) = yd - l_j1j2*cos(psi1)*psi1d - l_j2j3*cos(psi2)*psi2d;
va1 = zeros(2, 8);
va2 = zeros(2, 8);
psidj = [psi1d, psi2d, psi3d]';
for i = 1:8
    va1(:, i) = [vxj(IU(i)); vyj(IU(i))] - n(:, IU(i))*l_ja(i)*psidj(IU(i)) + (-1)*u(:, IU(i))*ha(i)*psidj(IU(i));
    va2(:, i) = [vxj(IU(i)); vyj(IU(i))] - n(:, IU(i))*l_ja(i)*psidj(IU(i)) + u(:, IU(i))*ha(i)*psidj(IU(i));
end

va1_v = zeros(2, 8);
va2_v = zeros(2, 8);
for i = 1:8
    va1_v(:, i) = inv(Rot_w2v(:, :, IU(i)))*va1(:, i);
    va2_v(:, i) = inv(Rot_w2v(:, :, IU(i)))*va2(:, i);
end

beta_wv_y = zeros(3, 1);
beta_wv_y(1) = (-(xd*cos(psi1) - yd*sin(psi1))*sin(psi1) + (xd*sin(psi1) + yd*cos(psi1))*cos(psi1)) - (-xd * sin(psi1) + yd * cos(psi1));
beta_wv_y(2) = (-(xd*cos(psi1) - yd*sin(psi1))*sin(psi2) + (xd*sin(psi1) + yd*cos(psi1))*cos(psi2)) - (-xd * sin(psi2) + yd * cos(psi2));
beta_wv_y(3) = (-(xd*cos(psi1) - yd*sin(psi1))*sin(psi3) + (xd*sin(psi1) + yd*cos(psi1))*cos(psi3)) - (-xd * sin(psi3) + yd * cos(psi3));
beta_wv_x = zeros(3, 1);
beta_wv_x(1) = ((xd*cos(psi1) - yd*sin(psi1))*cos(psi1) + (xd*sin(psi1) + yd*cos(psi1))*sin(psi1)) - (xd * cos(psi1) + yd * sin(psi1));
beta_wv_x(2) = ((xd*cos(psi1) - yd*sin(psi1))*cos(psi2) + (xd*sin(psi1) + yd*cos(psi1))*sin(psi2)) - (xd * cos(psi2) + yd * sin(psi2));
beta_wv_x(3) = ((xd*cos(psi1) - yd*sin(psi1))*cos(psi3) + (xd*sin(psi1) + yd*cos(psi1))*sin(psi3)) - (xd * cos(psi3) + yd * sin(psi3));

beta1 = zeros(8, 1);
beta2 = zeros(8, 1);
for i = 1:8
    beta1(i) = atan2(va1_v(2, i) + beta_wv_y(IU(i)), va1_v(1, i) + beta_wv_x(IU(i)));
    beta2(i) = atan2(va2_v(2, i) + beta_wv_y(IU(i)), va2_v(1, i) + beta_wv_x(IU(i)));
end

ca = [ca1, ca2, ca3, ca4, ca5, ca6, ca7, ca8]';
Ca = diag(ca);

Tau_tire = L_long1 * (- Delta_s * Ca * (delta - beta1)) ...
         + L_long2 * (- Delta_s * Ca * (delta - beta2)) ...
         + L_lat1 * (Delta_c * Ca * (delta - beta1)) ...
         + L_lat2 * (Delta_c * Ca * (delta - beta2));

Tau_tire = Twv' * Tau_tire;

beta = (beta1 + beta2) / 2;
Alpha = delta - beta;

end

== matlab function f_validation_V1_19b/time-domain-test/double-general-lineartyre-nonlinear-constant-matrix/Twv ==
  data: q input; qd input; Twv output; Tdwv output
function [Twv, Tdwv] = w2v(q, qd)

psi1 = q(3);
psi1d = qd(3);

Twv = [cos(psi1), -sin(psi1), 0, 0, 0;
     sin(psi1), cos(psi1), 0, 0, 0;
     0, 0, 1, 0, 0;
     0, 0, 0, 1, 0;
     0, 0, 0, 0, 1;];

Tdwv = [-sin(psi1)*psi1d, -cos(psi1)*psi1d, 0, 0, 0;
        cos(psi1)*psi1d, -sin(psi1)*psi1d, 0, 0, 0;
        0, 0, 0, 0, 0;
        0, 0, 0, 0, 0;
        0, 0, 0, 0, 0;];

end

== matlab function f_validation_V1_19b/time-domain-test/double-general-lineartyre-nonlinear-constant-matrix/qdd ==
  data: qd_v input; qdd_v input; qdd_n output; Twv input; Tdwv input
function qdd_n = qdd_v2w(qd_v, qdd_v, Twv, Tdwv)

qdd_n = Twv * qdd_v + Tdwv * qd_v;

end

== matlab function f_validation_V1_19b/time-domain-test/double-general-lineartyre-nonlinear-constant-matrix/qdd_v ==
  data: Mv input; Cv input; Dv input; Qv input; qd_v input; qdd_v output
function qdd_v = calculate_qdd(Mv, Cv, Dv, Qv, qd_v)

qdd_v = inv(Mv)*(Qv - Cv * qd_v - Dv * qd_v);

qdd_v(1) = 0;

end

== matlab function f_validation_V1_19b/time-domain-test/double-general-lineartyre-nonlinear-constant-matrix/w2v ==
  data: q input; qd input; q_v output; qd_v output
function [q_v, qd_v] = w2v(q, qd)

x = q(1);
y = q(2);
psi1 = q(3);

v_Rot_w = [cos(psi1), sin(psi1);
           -sin(psi1), cos(psi1)];

w_T_v = [cos(psi1), -sin(psi1), 0, 0, 0;
       sin(psi1), cos(psi1), 0, 0, 0;
       0, 0, 1, 0, 0;
       0, 0, 0, 1, 0;
       0, 0, 0, 0, 1;];

q_v = zeros(5, 1);
qd_v = zeros(5, 1);

q_v(1:2, :) = v_Rot_w * [x; y];
q_v(3:5, :) = q(3:5, :);

qd_v = inv(w_T_v) * qd;

end

== matlab function f_validation_V1_19b/time-domain-test/double-general-nonlineartyre-nonlinear-constant-matrix/C ==
  data: q input; qd input; C output
function C = calculate_C(q, qd)

m1 = 11142;
m3 = 11142;
m2 = 7651; 
l_j1j2 = 11.4;
l_j2j3 = 9.4;
l_j1g1 = 5.862; 
l_j2g2 = 4.643; 
l_j3g3 = 5.538; 

psi1 = q(3);
psi2 = q(4);
psi3 = q(5);
xd = qd(1);
yd = qd(2);
psi1d = qd(3);
psi2d = qd(4);
psi3d = qd(5);

C = [0, 0, (l_j1g1*m1 + l_j1j2*(m2 + m3))*cos(psi1)*psi1d, (l_j2g2*m2 + l_j2j3*m3)*cos(psi2)*psi2d, l_j3g3*m3*cos(psi3)*psi3d;
     0, 0, (l_j1g1*m1 + l_j1j2*(m2 + m3))*sin(psi1)*psi1d, (l_j2g2*m2 + l_j2j3*m3)*sin(psi2)*psi2d, l_j3g3*m3*sin(psi3)*psi3d;
     1/2*(l_j1g1*m1 + l_j1j2*(m2 + m3))*cos(psi1)*psi1d, 1/2*(l_j1g1*m1 + l_j1j2*(m2 + m3))*sin(psi1)*psi1d, -1/2*(l_j1g1*m1 + l_j1j2*(m2 + m3))*(xd*cos(psi1)+yd*sin(psi1))+1/2*(l_j2g2*l_j1j2*m2+l_j1j2*l_j2j3*m3)*sin(psi1-psi2)*psi2d+1/2*l_j3g3*l_j1j2*m3*sin(psi1-psi3)*psi3d, (l_j2g2*l_j1j2*m2+l_j1j2*l_j2j3*m3)*sin(psi1-psi2)*(-1/2*psi1d+psi2d), l_j3g3*l_j1j2*m3*sin(psi1-psi3)*(-1/2*psi1d+psi3d);
     1/2*(l_j2g2*m2 + l_j2j3*m3)*cos(psi2)*psi2d, 1/2*(l_j2g2*m2 + l_j2j3*m3)*sin(psi2)*psi2d, (l_j2g2*l_j1j2*m2+l_j1j2*l_j2j3*m3)*sin(psi1-psi2)*(-psi1d+1/2*psi2d), -1/2*(l_j2g2*m2+l_j2j3*m3)*(xd*cos(psi2)+yd*sin(psi2))-1/2*(l_j2g2*l_j1j2*m2+l_j1j2*l_j2j3*m3)*sin(psi1-psi2)*psi1d+1/2*l_j3g3*l_j2j3*m3*sin(psi2-psi3)*psi3d, l_j3g3*l_j2j3*m3*sin(psi2-psi3)*(-1/2*psi2d+psi3d);
     1/2*l_j3g3*m3*cos(psi3)*psi3d, 1/2*l_j3g3*m3*sin(psi3)*psi3d, l_j3g3*l_j1j2*m3*sin(psi1-psi3)*(-psi1d+1/2*psi3d), l_j3g3*l_j2j3*m3*sin(psi2-psi3)*(-psi2d+1/2*psi3d), -1/2*l_j3g3*m3*(xd*cos(psi3)+yd*sin(psi3))-1/2*l_j3g3*l_j1j2*m3*sin(psi1-psi3)*psi1d-1/2*l_j3g3*l_j2j3*m3*sin(psi2-psi3)*psi2d;];

c33 = -1/2*(l_j1g1*m1 + l_j1j2*(m2 + m3)) * ( (xd*cos(psi1)-yd*sin(psi1)-xd) * cos(psi1) + (xd*sin(psi1)+yd*cos(psi1)-yd) * sin(psi1) );
c44 = -1/2*(l_j2g2*m2 + l_j2j3*m3) * ( (xd*cos(psi1)-yd*sin(psi1)-xd) * cos(psi2) + (xd*sin(psi1)+yd*cos(psi1)-yd) * sin(psi2) );
c55 = -1/2*l_j3g3*m3 * ( (xd*cos(psi1)-yd*sin(psi1)-xd) * cos(psi3) + (xd*sin(psi1)+yd*cos(psi1)-yd) * sin(psi3) );
C_wv = [0, 0, 0, 0, 0;
        0, 0 ,0, 0, 0;
        0, 0, c33, 0, 0;
        0, 0, 0, c44, 0;
        0, 0, 0, 0, c55;];

C = C + C_wv;

end

== matlab function f_validation_V1_19b/time-domain-test/double-general-nonlineartyre-nonlinear-constant-matrix/Cv ==
  data: M input; C input; Cv output; Twv input; Tdwv input
function Cv = calculate_Mv(M, C, Twv, Tdwv)

Cv = Twv'*C*Twv + Twv'*M*Tdwv;

end

== matlab function f_validation_V1_19b/time-domain-test/double-general-nonlineartyre-nonlinear-constant-matrix/D ==
  data: D output
function D = calculate_D()

d1 = 10000;
d2 = 10000;

delta_kj = eye(3);
dj = [0, d1, d2, 0]';
D = zeros(5);

for k = 1:5
    for l = 1:5
        if k > 2 && l > 2
            if  l == k
                D(k, l) = (1 - delta_kj(1, k-2))*dj(k - 2) + (1 - delta_kj(3, k-2))*dj(k - 1);
            elseif l == k-1
                D(k, l) = -(1 - delta_kj(1, k-2))*dj(k - 2);
            elseif l == k+1
                D(k, l) = -(1 - delta_kj(3, k-2))*dj(k - 1);
            else
                D(k, l) = 0;
            end
        end
    end
end

end

== matlab function f_validation_V1_19b/time-domain-test/double-general-nonlineartyre-nonlinear-constant-matrix/Dv ==
  data: D input; Dv output; Twv input
function Dv = calculate_Mv(D, Twv)

Dv = Twv'*D*Twv;

end

== matlab function f_validation_V1_19b/time-domain-test/double-general-nonlineartyre-nonlinear-constant-matrix/M ==
  data: M output; q input
function M = calculate_M(q)

psi1 = q(3);
psi2 = q(4);
psi3 = q(5);

m1 = 11142;
m3 = 11142;
m2 = 7651; 
l_j1j2 = 11.4;
l_j2j3 = 9.4;
l_j1g1 = 5.862; 
l_j2g2 = 4.643; 
l_j3g3 = 5.538; 
iz1 = 143570; 
iz3 = 143570; 
iz2 = 37800;

l_kj = [l_j1g1, l_j1j2, l_j1j2;
             0, l_j2g2, l_j2j3;
             0,      0, l_j3g3;];
delta_kj = eye(3);
Jc = zeros(3, 5, 3);
for j = 1:3
    Jc(:, :, j) = [1, 0,  l_kj(1, j) * sin(psi1),  l_kj(2, j) * sin(psi2),  l_kj(3, j) * sin(psi3);
          0, 1, -l_kj(1, j) * cos(psi1), -l_kj(2, j) * cos(psi2), -l_kj(3, j) * cos(psi3);
          0, 0,          delta_kj(1, j),          delta_kj(2, j),          delta_kj(3, j);];
end

mj = [m1, m2, m3]';
izj = [iz1, iz2, iz3]';
Mj = zeros(3, 3, 3);
for j = 1:3
    Mj(:, :, j) = diag([mj(j), mj(j), izj(j)]);
end

M = zeros(5, 5);
for j = 1:3
    M = M + Jc(:, :, j)' * Mj(:, :, j) * Jc(:, :, j);
end

end

== matlab function f_validation_V1_19b/time-domain-test/double-general-nonlineartyre-nonlinear-constant-matrix/Mv ==
  data: M input; Mv output; Twv input
function Mv = calculate_Mv(M, Twv)

Mv = Twv'*M*Twv;

end

== matlab function f_validation_V1_19b/time-domain-test/double-general-nonlineartyre-nonlinear-constant-matrix/Tau_tire_v ==
  data: Tau_tire output; Alpha output; q input; qd input; Twv input; delta input
function [Tau_tire, Alpha] = calculate_Tau_tire(q, qd, Twv, delta)

% coefficient

l_j1j2 = 11.4;
l_j2j3 = 9.4;
l_j1a1 = 2.5;
l_j1a2 = 4;
l_j1a3 = 9.9;
l_j2a4 = 1.5;
l_j2a5 = 7.9;
l_j3a6 = 1.5;
l_j3a7 = 7.4;
l_j3a8 = 8.9;
h11 = 0.9625;
h12 = 0.9625;
h13 = 0.98;
h21 = 0.98; 
h22 = 0.98;
h31 = 0.98;
h32 = 0.9625;
h33 = 0.9625;

x = q(1);
y = q(2);
psi1 = q(3);
psi2 = q(4);
psi3 = q(5);
xd = qd(1);
yd = qd(2);
psi1d = qd(3);
psi2d = qd(4);
psi3d = qd(5);

psij = [psi1, psi2, psi3]';
Rot_w2v = zeros(2, 2, 3);
for i = 1:3
    Rot_w2v(:, :, i) = [cos(psij(i)), -sin(psij(i));
                        sin(psij(i)), cos(psij(i));];
end

Rot_v2t = zeros(2, 2, 8);
for i = 1:8
    Rot_v2t(:, :, i) = [cos(delta(i)), -sin(delta(i));
                        sin(delta(i)), cos(delta(i));];
end

xj = zeros(3, 1);
yj = zeros(3, 1);
xj(1) = x;
yj(1) = y;
xj(2) = x - l_j1j2*cos(psi1);
yj(2) = y - l_j1j2*sin(psi1);
xj(3) = x - l_j1j2*cos(psi1) - l_j2j3*cos(psi2);
yj(3) = y - l_j1j2*sin(psi1) - l_j2j3*sin(psi2);

u = zeros(2, 3);
n = zeros(2, 3);
for i = 1:3
    u(:, i)=[cos(q(i + 2)), sin(q(i + 2))]';
    n(:, i)=[-sin(q(i + 2)), cos(q(i + 2))]';
end

IU = [1, 1, 1, 2, 2, 3, 3, 3]';
l_ja = [l_j1a1, l_j1a2, l_j1a3, l_j2a4, l_j2a5, l_j3a6, l_j3a7, l_j3a8]';
ha = [h11, h12, h13, h21, h22, h31, h32, h33]';

L_long1 = [cos(psi1), cos(psi1), cos(psi1), cos(psi2), cos(psi2), cos(psi3), cos(psi3), cos(psi3);
           sin(psi1), sin(psi1), sin(psi1), sin(psi2), sin(psi2), sin(psi3), sin(psi3), sin(psi3);
           -h11, -h12, -h13, l_j1j2*sin(psi1-psi2), l_j1j2*sin(psi1-psi2), l_j1j2*sin(psi1-psi3), l_j1j2*sin(psi1-psi3), l_j1j2*sin(psi1-psi3);
           0, 0, 0, -h21, -h22, l_j2j3*sin(psi2-psi3), l_j2j3*sin(psi2-psi3), l_j2j3*sin(psi2-psi3);
           0, 0, 0, 0, 0, -h31, -h32, -h33;];

L_long2 = [cos(psi1), cos(psi1), cos(psi1), cos(psi2), cos(psi2), cos(psi3), cos(psi3), cos(psi3);
           sin(psi1), sin(psi1), sin(psi1), sin(psi2), sin(psi2), sin(psi3), sin(psi3), sin(psi3);
           h11, h12, h13, l_j1j2*sin(psi1-psi2), l_j1j2*sin(psi1-psi2), l_j1j2*sin(psi1-psi3), l_j1j2*sin(psi1-psi3), l_j1j2*sin(psi1-psi3);
           0, 0, 0, h21, h22, l_j2j3*sin(psi2-psi3), l_j2j3*sin(psi2-psi3), l_j2j3*sin(psi2-psi3);
           0, 0, 0, 0, 0, h31, h32, h33;];

L_lat1 = [-sin(psi1), -sin(psi1), -sin(psi1), -sin(psi2), -sin(psi2), -sin(psi3), -sin(psi3), -sin(psi3);
          cos(psi1), cos(psi1), cos(psi1), cos(psi2), cos(psi2), cos(psi3), cos(psi3), cos(psi3);
          -l_j1a1, -l_j1a2, -l_j1a3, -l_j1j2*cos(psi1-psi2), -l_j1j2*cos(psi1-psi2), -l_j1j2*cos(psi1-psi3), -l_j1j2*cos(psi1-psi3), -l_j1j2*cos(psi1-psi3);
          0, 0, 0, -l_j2a4, -l_j2a5, -l_j2j3*cos(psi2-psi3), -l_j2j3*cos(psi2-psi3), -l_j2j3*cos(psi2-psi3);
          0, 0, 0, 0, 0, -l_j3a6, -l_j3a7, -l_j3a8;];

L_lat2 = [-sin(psi1), -sin(psi1), -sin(psi1), -sin(psi2), -sin(psi2), -sin(psi3), -sin(psi3), -sin(psi3);
          cos(psi1), cos(psi1), cos(psi1), cos(psi2), cos(psi2), cos(psi3), cos(psi3), cos(psi3);
          -l_j1a1, -l_j1a2, -l_j1a3, -l_j1j2*cos(psi1-psi2), -l_j1j2*cos(psi1-psi2), -l_j1j2*cos(psi1-psi3), -l_j1j2*cos(psi1-psi3), -l_j1j2*cos(psi1-psi3);
          0, 0, 0, -l_j2a4, -l_j2a5, -l_j2j3*cos(psi2-psi3), -l_j2j3*cos(psi2-psi3), -l_j2j3*cos(psi2-psi3);
          0, 0, 0, 0, 0, -l_j3a6, -l_j3a7, -l_j3a8;];

Delta_c = zeros(8, 8);
Delta_s = zeros(8, 8);
for i = 1:8
    Delta_c(i, i) = cos(delta(i));
    Delta_s(i, i) = sin(delta(i));
end

vxj = zeros(3, 1);
vyj = zeros(3, 1);
vxj(1) = xd;
vyj(1) = yd;
vxj(2) = xd + l_j1j2*sin(psi1)*psi1d;
vyj(2) = yd - l_j1j2*cos(psi1)*psi1d;
vxj(3) = xd + l_j1j2*sin(psi1)*psi1d + l_j2j3*sin(psi2)*psi2d;
vyj(3) = yd - l_j1j2*cos(psi1)*psi1d - l_j2j3*cos(psi2)*psi2d;
va1 = zeros(2, 8);
va2 = zeros(2, 8);
psidj = [psi1d, psi2d, psi3d]';
for i = 1:8
    va1(:, i) = [vxj(IU(i)); vyj(IU(i))] - n(:, IU(i))*l_ja(i)*psidj(IU(i)) + (-1)*u(:, IU(i))*ha(i)*psidj(IU(i));
    va2(:, i) = [vxj(IU(i)); vyj(IU(i))] - n(:, IU(i))*l_ja(i)*psidj(IU(i)) + u(:, IU(i))*ha(i)*psidj(IU(i));
end

va1_v = zeros(2, 8);
va2_v = zeros(2, 8);
for i = 1:8
    va1_v(:, i) = inv(Rot_w2v(:, :, IU(i)))*va1(:, i);
    va2_v(:, i) = inv(Rot_w2v(:, :, IU(i)))*va2(:, i);
end

beta_wv_y = zeros(3, 1);
beta_wv_y(1) = (-(xd*cos(psi1) - yd*sin(psi1))*sin(psi1) + (xd*sin(psi1) + yd*cos(psi1))*cos(psi1)) - (-xd * sin(psi1) + yd * cos(psi1));
beta_wv_y(2) = (-(xd*cos(psi1) - yd*sin(psi1))*sin(psi2) + (xd*sin(psi1) + yd*cos(psi1))*cos(psi2)) - (-xd * sin(psi2) + yd * cos(psi2));
beta_wv_y(3) = (-(xd*cos(psi1) - yd*sin(psi1))*sin(psi3) + (xd*sin(psi1) + yd*cos(psi1))*cos(psi3)) - (-xd * sin(psi3) + yd * cos(psi3));
beta_wv_x = zeros(3, 1);
beta_wv_x(1) = ((xd*cos(psi1) - yd*sin(psi1))*cos(psi1) + (xd*sin(psi1) + yd*cos(psi1))*sin(psi1)) - (xd * cos(psi1) + yd * sin(psi1));
beta_wv_x(2) = ((xd*cos(psi1) - yd*sin(psi1))*cos(psi2) + (xd*sin(psi1) + yd*cos(psi1))*sin(psi2)) - (xd * cos(psi2) + yd * sin(psi2));
beta_wv_x(3) = ((xd*cos(psi1) - yd*sin(psi1))*cos(psi3) + (xd*sin(psi1) + yd*cos(psi1))*sin(psi3)) - (xd * cos(psi3) + yd * sin(psi3));

beta1 = zeros(8, 1);
beta2 = zeros(8, 1);
for i = 1:8
    beta1(i) = atan2(va1_v(2, i) + beta_wv_y(IU(i)), va1_v(1, i) + beta_wv_x(IU(i)));
    beta2(i) = atan2(va2_v(2, i) + beta_wv_y(IU(i)), va2_v(1, i) + beta_wv_x(IU(i)));
end

% magic formula

% 魔术公式参数
A = [1.65, -34, 1250, 4535, 12.8, 0.00501, -0.02103,  0.77394, ...
     0.0022890, 0.013442, 0.003709, 19.1656, 1.21356, 6.26206]';

% 轮胎垂向载荷 kN
Fz = 30000 / 1000;

Fy1 = zeros(8, 1);
Fy2 = zeros(8, 1);
gamma = 0;
for i = 1:8
    alpha = (delta(i) - beta1(i)) * 180 / pi;
    Sh = A(10) * Fz + A(11) + A(9) * gamma;
    Sv = A(12) * Fz * gamma + A(13) * Fz + A(14);
    C = A(1);
    D = A(2) * Fz ^ 2 + A(3) * Fz;
    BCD = A(4) * sin(2 * atan(Fz / A(5))) * (1 - A(6) * abs(gamma));
    B = BCD / (C * D);
    E = A(7) * Fz + A(8);
    x = alpha; % + Sh;
    % 轮胎侧向力
    Fy1(i) = D * sin(C * atan(B * x - E * (B * x - atan(B * x)))); % + Sv;
end
for i = 1:8
    alpha = (delta(i) - beta2(i)) * 180 / pi;
    Sh = A(10) * Fz + A(11) + A(9) * gamma;
    Sv = A(12) * Fz * gamma + A(13) * Fz + A(14);
    C = A(1);
    D = A(2) * Fz ^ 2 + A(3) * Fz;
    BCD = A(4) * sin(2 * atan(Fz / A(5))) * (1 - A(6) * abs(gamma));
    B = BCD / (C * D);
    E = A(7) * Fz + A(8);
    x = alpha; % + Sh;
    % 轮胎侧向力
    Fy2(i) = D * sin(C * atan(B * x - E * (B * x - atan(B * x)))); % + Sv;
end

Tau_tire = L_long1 * (- Delta_s * Fy1) ...
         + L_long2 * (- Delta_s * Fy2) ...
         + L_lat1 * (Delta_c * Fy1) ...
         + L_lat2 * (Delta_c * Fy2);

Tau_tire = Twv' * Tau_tire;

beta = (beta1 + beta2) / 2;
Alpha = delta - beta;

end

== matlab function f_validation_V1_19b/time-domain-test/double-general-nonlineartyre-nonlinear-constant-matrix/Twv ==
  data: q input; qd input; Twv output; Tdwv output
function [Twv, Tdwv] = w2v(q, qd)

psi1 = q(3);
psi1d = qd(3);

Twv = [cos(psi1), -sin(psi1), 0, 0, 0;
     sin(psi1), cos(psi1), 0, 0, 0;
     0, 0, 1, 0, 0;
     0, 0, 0, 1, 0;
     0, 0, 0, 0, 1;];

Tdwv = [-sin(psi1)*psi1d, -cos(psi1)*psi1d, 0, 0, 0;
        cos(psi1)*psi1d, -sin(psi1)*psi1d, 0, 0, 0;
        0, 0, 0, 0, 0;
        0, 0, 0, 0, 0;
        0, 0, 0, 0, 0;];

end

== matlab function f_validation_V1_19b/time-domain-test/double-general-nonlineartyre-nonlinear-constant-matrix/qdd ==
  data: qd_v input; qdd_v input; qdd_n output; Twv input; Tdwv input
function qdd_n = qdd_v2w(qd_v, qdd_v, Twv, Tdwv)

qdd_n = Twv * qdd_v + Tdwv * qd_v;

end

== matlab function f_validation_V1_19b/time-domain-test/double-general-nonlineartyre-nonlinear-constant-matrix/qdd_v ==
  data: Mv input; Cv input; Dv input; Qv input; qd_v input; qdd_v output
function qdd_v = calculate_qdd(Mv, Cv, Dv, Qv, qd_v)

qdd_v = inv(Mv)*(Qv - Cv * qd_v - Dv * qd_v);

qdd_v(1) = 0;

end

== matlab function f_validation_V1_19b/time-domain-test/double-general-nonlineartyre-nonlinear-constant-matrix/w2v ==
  data: q input; qd input; q_v output; qd_v output
function [q_v, qd_v] = w2v(q, qd)

x = q(1);
y = q(2);
psi1 = q(3);

v_Rot_w = [cos(psi1), sin(psi1);
           -sin(psi1), cos(psi1)];

w_T_v = [cos(psi1), -sin(psi1), 0, 0, 0;
       sin(psi1), cos(psi1), 0, 0, 0;
       0, 0, 1, 0, 0;
       0, 0, 0, 1, 0;
       0, 0, 0, 0, 1;];

q_v = zeros(5, 1);
qd_v = zeros(5, 1);

q_v(1:2, :) = v_Rot_w * [x; y];
q_v(3:5, :) = q(3:5, :);

qd_v = inv(w_T_v) * qd;

end

== matlab function f_validation_V1_19b/time-domain-test/double-general-nonlineartyre-nonlinear-variable-matrix/C ==
  data: q input; qd input; C output
function C = calculate_C(q, qd)

m1 = 11142;
m3 = 11142;
m2 = 7651; 
l_j1j2 = 11.4;
l_j2j3 = 9.4;
l_j1g1 = 5.862; 
l_j2g2 = 4.643; 
l_j3g3 = 5.538; 

psi1 = q(3);
psi2 = q(4);
psi3 = q(5);
xd = qd(1);
yd = qd(2);
psi1d = qd(3);
psi2d = qd(4);
psi3d = qd(5);

C = [0, 0, (l_j1g1*m1 + l_j1j2*(m2 + m3))*cos(psi1)*psi1d, (l_j2g2*m2 + l_j2j3*m3)*cos(psi2)*psi2d, l_j3g3*m3*cos(psi3)*psi3d;
     0, 0, (l_j1g1*m1 + l_j1j2*(m2 + m3))*sin(psi1)*psi1d, (l_j2g2*m2 + l_j2j3*m3)*sin(psi2)*psi2d, l_j3g3*m3*sin(psi3)*psi3d;
     1/2*(l_j1g1*m1 + l_j1j2*(m2 + m3))*cos(psi1)*psi1d, 1/2*(l_j1g1*m1 + l_j1j2*(m2 + m3))*sin(psi1)*psi1d, -1/2*(l_j1g1*m1 + l_j1j2*(m2 + m3))*(xd*cos(psi1)+yd*sin(psi1))+1/2*(l_j2g2*l_j1j2*m2+l_j1j2*l_j2j3*m3)*sin(psi1-psi2)*psi2d+1/2*l_j3g3*l_j1j2*m3*sin(psi1-psi3)*psi3d, (l_j2g2*l_j1j2*m2+l_j1j2*l_j2j3*m3)*sin(psi1-psi2)*(-1/2*psi1d+psi2d), l_j3g3*l_j1j2*m3*sin(psi1-psi3)*(-1/2*psi1d+psi3d);
     1/2*(l_j2g2*m2 + l_j2j3*m3)*cos(psi2)*psi2d, 1/2*(l_j2g2*m2 + l_j2j3*m3)*sin(psi2)*psi2d, (l_j2g2*l_j1j2*m2+l_j1j2*l_j2j3*m3)*sin(psi1-psi2)*(-psi1d+1/2*psi2d), -1/2*(l_j2g2*m2+l_j2j3*m3)*(xd*cos(psi2)+yd*sin(psi2))-1/2*(l_j2g2*l_j1j2*m2+l_j1j2*l_j2j3*m3)*sin(psi1-psi2)*psi1d+1/2*l_j3g3*l_j2j3*m3*sin(psi2-psi3)*psi3d, l_j3g3*l_j2j3*m3*sin(psi2-psi3)*(-1/2*psi2d+psi3d);
     1/2*l_j3g3*m3*cos(psi3)*psi3d, 1/2*l_j3g3*m3*sin(psi3)*psi3d, l_j3g3*l_j1j2*m3*sin(psi1-psi3)*(-psi1d+1/2*psi3d), l_j3g3*l_j2j3*m3*sin(psi2-psi3)*(-psi2d+1/2*psi3d), -1/2*l_j3g3*m3*(xd*cos(psi3)+yd*sin(psi3))-1/2*l_j3g3*l_j1j2*m3*sin(psi1-psi3)*psi1d-1/2*l_j3g3*l_j2j3*m3*sin(psi2-psi3)*psi2d;];

end

== matlab function f_validation_V1_19b/time-domain-test/double-general-nonlineartyre-nonlinear-variable-matrix/D ==
  data: D output
function D = calculate_D()

d1 = 10000;
d2 = 10000;

delta_kj = eye(3);
dj = [0, d1, d2, 0]';
D = zeros(5);

for k = 1:5
    for l = 1:5
        if k > 2 && l > 2
            if  l == k
                D(k, l) = (1 - delta_kj(1, k-2))*dj(k - 2) + (1 - delta_kj(3, k-2))*dj(k - 1);
            elseif l == k-1
                D(k, l) = -(1 - delta_kj(1, k-2))*dj(k - 2);
            elseif l == k+1
                D(k, l) = -(1 - delta_kj(3, k-2))*dj(k - 1);
            else
                D(k, l) = 0;
            end
        end
    end
end

end

== matlab function f_validation_V1_19b/time-domain-test/double-general-nonlineartyre-nonlinear-variable-matrix/M ==
  data: M output; q input
function M = calculate_M(q)

psi1 = q(3);
psi2 = q(4);
psi3 = q(5);

m1 = 11142;
m3 = 11142;
m2 = 7651; 
l_j1j2 = 11.4;
l_j2j3 = 9.4;
l_j1g1 = 5.862; 
l_j2g2 = 4.643; 
l_j3g3 = 5.538; 
iz1 = 143570; 
iz3 = 143570; 
iz2 = 37800;

l_kj = [l_j1g1, l_j1j2, l_j1j2;
             0, l_j2g2, l_j2j3;
             0,      0, l_j3g3;];
delta_kj = eye(3);
Jc = zeros(3, 5, 3);
for j = 1:3
    Jc(:, :, j) = [1, 0,  l_kj(1, j) * sin(psi1),  l_kj(2, j) * sin(psi2),  l_kj(3, j) * sin(psi3);
          0, 1, -l_kj(1, j) * cos(psi1), -l_kj(2, j) * cos(psi2), -l_kj(3, j) * cos(psi3);
          0, 0,          delta_kj(1, j),          delta_kj(2, j),          delta_kj(3, j);];
end

mj = [m1, m2, m3]';
izj = [iz1, iz2, iz3]';
Mj = zeros(3, 3, 3);
for j = 1:3
    Mj(:, :, j) = diag([mj(j), mj(j), izj(j)]);
end

M = zeros(5, 5);
for j = 1:3
    M = M + Jc(:, :, j)' * Mj(:, :, j) * Jc(:, :, j);
end

end
